simulink model "Seesaw_PP"  (R2025b)
settings: Solver=ode4  StartTime=0.0  StopTime=10  FixedStep=0.001  RelTol=1e-3
undefined symbols (not defined in the file or in its folder): A_sw, B_sw, C_sw, D_sw, HIL, Kf, theta0
libraries: quarc_library x4
settings Model: Creator=U448565  LastModifiedBy=U448565

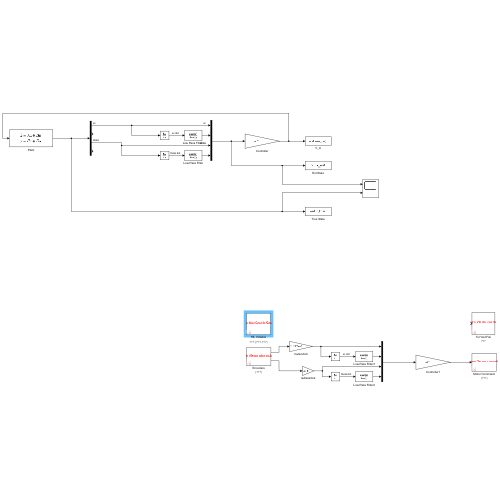
[thumbnail: Simulink's stored preview of the top-level diagram]
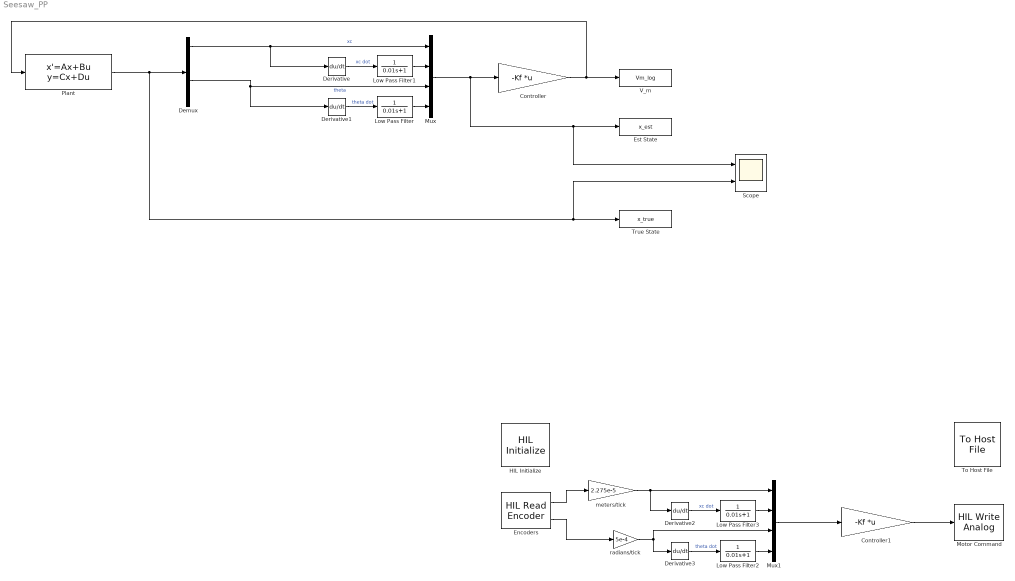
== system Seesaw_PP ==
  Controller : Gain  Gain=-Kf  Multiplication=Matrix(K*u)
  Controller1 : Gain  Gain=-Kf  Multiplication=Matrix(K*u)
  Demux : Demux
  Derivative{,1..3} (4 alike) : Derivative
  Encoders : quarc_library/Data Acquisition/Generic/Immediate I//O/HIL Read Encoder  object_name=HIL-1  channels=[0:1]  sample_time=qc_get_step_size  active=on  vector_output=off  data_type_mode=Inherit via back propagation  data_type=double
  Est State : ToWorkspace  VariableName=x_est  SaveFormat=Timeseries  SampleTime=-1
  HIL Initialize : quarc_library/Data Acquisition/Generic/Configuration/HIL Initialize  object_name=HIL-1  board_type=q2_usb  board_number=0  board_options=d0=digital;d1=digital;led=auto;update_rate=normal  exclusive=off  active=off  hardware_clocks=[0:2]  clock_modes=[]  initial_clock_frequencies=[]  set_clock_params_at_start=off  set_clock_params_at_switch_in=off  set_clock_frequencies_at_start=off  set_clock_frequencies_at_switch_in=off  analog_input_channels=[0:1]  analog_input_configurations=[]  analog_input_maximums=10  analog_input_minimums=-10  set_analog_input_params_at_start=on  set_analog_input_params_at_switch_in=off  analog_output_channels=[0:1]  analog_output_maximums=10  analog_output_minimums=-10  initial_analog_outputs=[0]  final_analog_outputs=[0]  watchdog_analog_outputs=0  set_analog_output_params_at_start=on  set_analog_output_params_at_switch_in=off  set_analog_outputs_at_start=on  set_analog_outputs_at_switch_in=off  set_analog_outputs_at_terminate=on  set_analog_outputs_at_switch_out=off  set_analog_outputs_on_watchdog=off  digital_input_channels=[]  digital_output_channels=[0:7]  digital_output_configuration=[]  initial_digital_outputs=[0]  final_digital_outputs=[0]  watchdog_digital_outputs=[0]  set_digital_output_params_at_start=off  set_digital_output_params_at_switch_in=off  set_digital_outputs_at_start=on  set_digital_outputs_at_switch_in=off  set_digital_outputs_at_terminate=on  set_digital_outputs_at_switch_out=off  set_digital_outputs_on_watchdog=off  encoder_channels=[0:1]  quadrature=[4]  encoder_filter_frequency=[]  initial_encoder_counts=[0]  set_encoder_params_at_start=on  set_encoder_params_at_switch_in=off  set_encoder_counts_at_start=on  set_encoder_counts_at_switch_in=off  pwm_channels=[]  pwm_modes=[0]  pwm_frequency=1/0.020  pwm_configuration=[]  pwm_alignment=[]  pwm_polarity=[]  pwm_leading_deadband=[]  pwm_trailing_deadband=[]  initial_pwm_outputs=[0]  final_pwm_outputs=[0]  watchdog_pwm_outputs=[0]  set_pwm_params_at_start=on  set_pwm_params_at_switch_in=off  set_pwm_outputs_at_start=on  set_pwm_outputs_at_switch_in=off  set_pwm_outputs_at_terminate=on  set_pwm_outputs_at_switch_out=off  set_pwm_outputs_on_watchdog=off  other_output_channels=[]  initial_other_outputs=[]  final_other_outputs=[]  watchdog_other_outputs=[]  set_other_outputs_at_start=off  set_other_outputs_at_switch_in=off  set_other_outputs_at_terminate=off  set_other_outputs_at_switch_out=off  set_other_outputs_on_watchdog=off
  Low Pass Filter{,1..3} (4 alike) : TransferFcn  Denominator=[0.01 1]
  Motor Command : quarc_library/Data Acquisition/Generic/Immediate I//O/HIL Write Analog  object_name=HIL-1  channels=0  sample_time=-1  active=off  vector_input=off
  Mux : Mux
  Mux1 : Mux
  Plant : StateSpace  A=A_sw  B=B_sw  C=C_sw  D=D_sw  InitialCondition=[0;0;theta0;0]
  Scope : Scope  NumInputPorts=2
      settings: ActiveDisplayYMinimum=-0.20814094676708719  ActiveDisplayYMaximum=0.56753923401338313
  To Host File : quarc_library/Sinks/To Host/To Host File  source=Specify via dialog (do not evaluate)  file_name=data_%{date}_%{time}.mat  variable_name=data  decimation=1  sample_time=-1  file_format=MAT-file v.4  options=No header or footer  append=off  final_file_name=data_05-Feb-2026_10-55-33.mat  encoding=Default  bitrate=0
  True State : ToWorkspace  VariableName=x_true  SaveFormat=Timeseries  SampleTime=-1
  V_m : ToWorkspace  VariableName=Vm_log  SaveFormat=Timeseries  SampleTime=-1
  meters/tick : Gain  Gain=2.275e-5
  radians/tick : Gain  Gain=5e-4
  wires:
  Plant/1 -> Demux/1, Scope/2, True State/1
  Demux/1 -> Derivative/1, Mux/1  "xc"
  Demux/3 -> Derivative1/1, Mux/3  "theta"
  Controller/1 -> Plant/1, V_m/1
  Derivative/1 -> Low Pass Filter1/1  "xc dot"
  Derivative1/1 -> Low Pass Filter/1  "theta dot"
  Mux/1 -> Controller/1, Scope/1, Est State/1
  Low Pass Filter/1 -> Mux/4
  Low Pass Filter1/1 -> Mux/2
  Derivative2/1 -> Low Pass Filter3/1  "xc dot"
  Low Pass Filter3/1 -> Mux1/2
  Low Pass Filter2/1 -> Mux1/4
  Mux1/1 -> Controller1/1
  Derivative3/1 -> Low Pass Filter2/1  "theta dot"
  Encoders/1 -> meters/tick/1
  Encoders/2 -> radians/tick/1
  meters/tick/1 -> Derivative2/1, Mux1/1
  radians/tick/1 -> Mux1/3, Derivative3/1
  Controller1/1 -> Motor Command/1
